simulink model "ofur"  (R2018b)
settings: Solver=VariableStepAuto  StartTime=0.0  StopTime=0.01  RelTol=1e-3
libraries: xbsIndex_r4 x105, commanapbnd3 x4
(part 2 of 2)

== matlab function ofur/MATLAB Function 1 ==
  data: u input; y output
function y = fcn(u)

persistent B
persistent D
persistent E
persistent C
persistent F
persistent n

persistent A,

A = [1 7 7 1 7 3 5 5];
%A = [1 1 1 0 1 0 1 1 1 0 0 1 0 0 0 0];

%A = [0.707 0.707 0.707 0.707 0.707 -0.707 -0.707 -0.707];

if isempty(B)
 B = 0;
end

if isempty(D)
 D = 0;
end

if isempty(C)
 C = 0;
end

if isempty(F)
 F = 0;
end

if isempty(E)
 E = 0;
end

if isempty(n)
 n = 1;
end
 
D = B;
B = u;

if B == 0 && D == 1
    E = 1;
else
    E = 0;
end

if E == 1
    if n < 8
        n = n + 1;
    else
        n = 1;
    end
    C = A(n);

end

y = C;

== matlab function ofur/MATLAB Function 3 ==
  data: u input; y output
function y = fcn(u)

persistent B
persistent D
persistent E
persistent C
persistent F
persistent n

persistent A,

A = [1 7 7 1 7 3 5 5];
%A = [1 1 1 0 1 0 1 1 1 0 0 1 0 0 0 0];

%A = [0.707 0.707 0.707 0.707 0.707 -0.707 -0.707 -0.707];

if isempty(B)
 B = 0;
end

if isempty(D)
 D = 0;
end

if isempty(C)
 C = 0;
end

if isempty(F)
 F = 0;
end

if isempty(E)
 E = 0;
end

if isempty(n)
 n = 1;
end
 
D = B;
B = u;

if B == 0 && D == 1
    E = 1;
else
    E = 0;
end

if E == 1
    if n < 8
        n = n + 1;
    else
        n = 1;
    end
    C = A(n);

end

y = C;

== matlab function ofur/MATLAB Function 2 ==
  data: u input; y output
function y = fcn(u)

persistent B
persistent D
persistent E
persistent C
persistent F
persistent n

persistent A,

A = [1 7 7 1 7 3 5 5];
%A = [1 1 1 0 1 0 1 1 1 0 0 1 0 0 0 0];

%A = [0.707 0.707 0.707 0.707 0.707 -0.707 -0.707 -0.707];

if isempty(B)
 B = 0;
end

if isempty(D)
 D = 0;
end

if isempty(C)
 C = 0;
end

if isempty(F)
 F = 0;
end

if isempty(E)
 E = 0;
end

if isempty(n)
 n = 1;
end
 
D = B;
B = u;

if B == 0 && D == 1
    E = 1;
else
    E = 0;
end

if E == 1
    if n < 8
        n = n + 1;
    else
        n = 1;
    end
    C = A(n);

end

y = C;
